simulink model "Karatsuba_Multiplier_64_Unsigned"  (R2012b)
settings: Solver=FixedStepDiscrete  SolverMode=SingleTasking  StartTime=0  StopTime=stopClock  RelTol=1e-3
libraries: xbsIndex_r4 x469
(part 1 of 3)
settings Model: Creator=UGG1  LastModifiedBy=UGG1

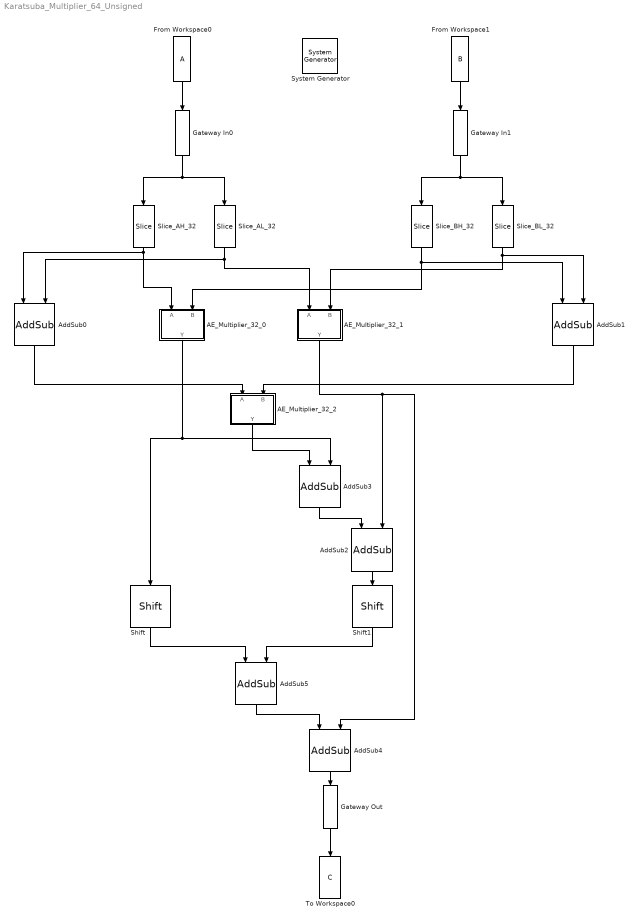
== system Karatsuba_Multiplier_64_Unsigned ==
  " System Generator" : xbsIndex_r4/ System Generator  Tag=genX  xilinxfamily=Kintex7  part=xc7k325t  speed=-3  package=fbg676  synthesis_tool=XST  clock_wrapper=Clock Enables  directory=./netlist  proj_type=Project Navigator  Synth_file=XST Defaults  Impl_file=ISE Defaults  testbench=off  simulink_period=1  sysclk_period=10  dcm_input_clock_period=10  incr_netlist=off  trim_vbits=Everywhere in SubSystem  dbl_ovrd=According to Block Masks  core_generation=According to Block Masks  run_coregen=off  deprecated_control=off  eval_field=0  block_type=sysgen
  AE_Multiplier_32_0 : Subsystem
  AE_Multiplier_32_1 : Subsystem
  AE_Multiplier_32_2 : Subsystem
  AddSub0 : xbsIndex_r4/AddSub  mode=Addition  use_carryin=off  use_carryout=off  en=off  latency=0  precision=User Defined  arith_type=Unsigned  n_bits=33  bin_pt=0  quantization=Truncate  overflow=Wrap  dbl_ovrd=off  use_behavioral_HDL=off  hw_selection=Fabric  pipelined=on  block_type=addsub
  AddSub1 : xbsIndex_r4/AddSub  mode=Addition  use_carryin=off  use_carryout=off  en=off  latency=0  precision=User Defined  arith_type=Unsigned  n_bits=33  bin_pt=0  quantization=Truncate  overflow=Wrap  dbl_ovrd=off  use_behavioral_HDL=off  hw_selection=Fabric  pipelined=on  block_type=addsub
  AddSub2 : xbsIndex_r4/AddSub  mode=Subtraction  use_carryin=off  use_carryout=off  en=off  latency=0  precision=User Defined  arith_type=Unsigned  n_bits=64  bin_pt=0  quantization=Truncate  overflow=Wrap  dbl_ovrd=off  use_behavioral_HDL=off  hw_selection=Fabric  pipelined=on  block_type=addsub
  AddSub3 : xbsIndex_r4/AddSub  mode=Subtraction  use_carryin=off  use_carryout=off  en=off  latency=0  precision=User Defined  arith_type=Unsigned  n_bits=64  bin_pt=0  quantization=Truncate  overflow=Wrap  dbl_ovrd=off  use_behavioral_HDL=off  hw_selection=Fabric  pipelined=on  block_type=addsub
  AddSub4 : xbsIndex_r4/AddSub  mode=Addition  use_carryin=off  use_carryout=off  en=off  latency=0  precision=User Defined  arith_type=Unsigned  n_bits=128  bin_pt=0  quantization=Truncate  overflow=Wrap  dbl_ovrd=off  use_behavioral_HDL=off  hw_selection=Fabric  pipelined=on  block_type=addsub
  AddSub5 : xbsIndex_r4/AddSub  mode=Addition  use_carryin=off  use_carryout=off  en=off  latency=0  precision=User Defined  arith_type=Unsigned  n_bits=128  bin_pt=0  quantization=Truncate  overflow=Wrap  dbl_ovrd=off  use_behavioral_HDL=off  hw_selection=Fabric  pipelined=on  block_type=addsub
  From Workspace0 : FromWorkspace  VariableName=A  SampleTime=0
  From Workspace1 : FromWorkspace  VariableName=B  SampleTime=0
  Gateway In0 : xbsIndex_r4/Gateway In  gui_display_data_type=Fixed-point  arith_type=Unsigned  n_bits=64  bin_pt=0  preci_type=Single  exp_width=8  frac_width=24  quantization="Round  (unbiased: +/- Inf)"  overflow=Saturate  period=1  dbl_ovrd=off  timing_constraint=None  locs_specified=off  LOCs={}  UseAsADC=off  ADCChannel='1'  inherit_from_input=off  hdl_port=on  block_type=gatewayin
  Gateway In1 : xbsIndex_r4/Gateway In  gui_display_data_type=Fixed-point  arith_type=Unsigned  n_bits=64  bin_pt=0  preci_type=Single  exp_width=8  frac_width=24  quantization="Round  (unbiased: +/- Inf)"  overflow=Saturate  period=1  dbl_ovrd=off  timing_constraint=None  locs_specified=off  LOCs={}  UseAsADC=off  ADCChannel='1'  inherit_from_input=off  hdl_port=on  block_type=gatewayin
  Gateway Out : xbsIndex_r4/Gateway Out  inherit_from_input=off  hdl_port=on  timing_constraint=None  locs_specified=off  LOCs={}  UseAsDAC=off  DACChannel='1'  block_type=gatewayout
  Shift : xbsIndex_r4/Shift  shift_dir=Left  shift_bits=64  en=off  latency=0  precision=User Defined  arith_type=Unsigned  n_bits=128  bin_pt=0  quantization=Truncate  overflow=Wrap  dbl_ovrd=off  block_type=shift
  Shift1 : xbsIndex_r4/Shift  shift_dir=Left  shift_bits=32  en=off  latency=0  precision=User Defined  arith_type=Unsigned  n_bits=128  bin_pt=0  quantization=Truncate  overflow=Wrap  dbl_ovrd=off  block_type=shift
  Slice_AH_32 : xbsIndex_r4/Slice  nbits=32  boolean_output=off  mode=Lower Bit Location + Width  bit1=0  base1=MSB of Input  bit0=32  base0=LSB of Input  dbl_ovrd=off  block_type=slice
  Slice_AL_32 : xbsIndex_r4/Slice  nbits=32  boolean_output=off  mode=Lower Bit Location + Width  bit1=0  base1=MSB of Input  bit0=0  base0=LSB of Input  dbl_ovrd=off  block_type=slice
  Slice_BH_32 : xbsIndex_r4/Slice  nbits=32  boolean_output=off  mode=Lower Bit Location + Width  bit1=0  base1=MSB of Input  bit0=32  base0=LSB of Input  dbl_ovrd=off  block_type=slice
  Slice_BL_32 : xbsIndex_r4/Slice  nbits=32  boolean_output=off  mode=Lower Bit Location + Width  bit1=0  base1=MSB of Input  bit0=0  base0=LSB of Input  dbl_ovrd=off  block_type=slice
  To Workspace0 : ToWorkspace  VariableName=C  SampleTime=-1  SaveFormat=Timeseries
  wires:
  From Workspace1/1 -> Gateway In1/1
  Gateway Out/1 -> To Workspace0/1
  From Workspace0/1 -> Gateway In0/1
  Gateway In0/1 -> Slice_AL_32/1, Slice_AH_32/1
  Gateway In1/1 -> Slice_BL_32/1, Slice_BH_32/1
  Slice_AH_32/1 -> AE_Multiplier_32_0/1(A), AddSub0/1
  Slice_BH_32/1 -> AE_Multiplier_32_0/2(B), AddSub1/1
  Slice_BL_32/1 -> AddSub1/2, AE_Multiplier_32_1/2(B)
  Slice_AL_32/1 -> AddSub0/2, AE_Multiplier_32_1/1(A)
  AddSub0/1 -> AE_Multiplier_32_2/1(A)
  AddSub1/1 -> AE_Multiplier_32_2/2(B)
  AE_Multiplier_32_2/1(Y) -> AddSub3/1
  AE_Multiplier_32_0/1(Y) -> Shift/1, AddSub3/2
  AddSub3/1 -> AddSub2/1
  AE_Multiplier_32_1/1(Y) -> AddSub4/2, AddSub2/2
  AddSub2/1 -> Shift1/1
  Shift/1 -> AddSub5/1
  Shift1/1 -> AddSub5/2
  AddSub5/1 -> AddSub4/1
  AddSub4/1 -> Gateway Out/1

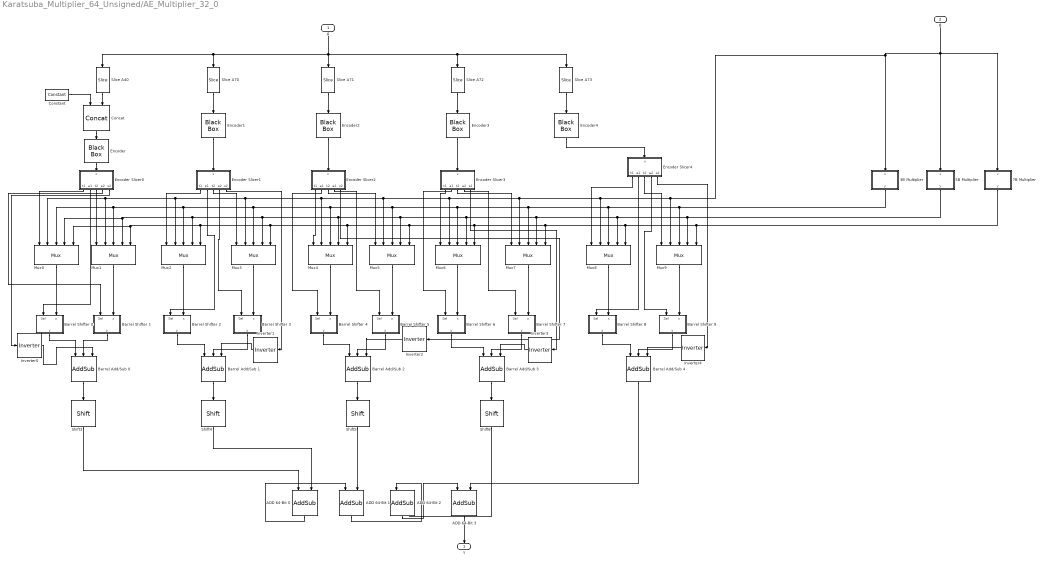
== system Karatsuba_Multiplier_64_Unsigned/AE_Multiplier_32_0 ==
  A : Inport
  B : Inport  Port=2
  3B Multiplier : Subsystem
  5B Multiplier : Subsystem
  7B Multiplier : Subsystem
  ADD 64-Bit {0..3} (4 alike) : xbsIndex_r4/AddSub  mode=Addition  use_carryin=off  use_carryout=off  en=off  latency=0  precision=User Defined  arith_type=Unsigned  n_bits=128  bin_pt=0  quantization=Truncate  overflow=Wrap  dbl_ovrd=off  use_behavioral_HDL=off  hw_selection=Fabric  pipelined=on  block_type=addsub
  Barrel Add/Sub {0..4} (5 alike) : xbsIndex_r4/AddSub  mode=Addition or Subtraction  use_carryin=off  use_carryout=off  en=off  latency=0  precision=User Defined  arith_type=Unsigned  n_bits=64  bin_pt=0  quantization=Truncate  overflow=Wrap  dbl_ovrd=off  use_behavioral_HDL=off  hw_selection=Fabric  pipelined=on  block_type=addsub
  Barrel Shifter 0 : Subsystem
  Barrel Shifter 1 : Subsystem
  Barrel Shifter 2 : Subsystem
  Barrel Shifter 3 : Subsystem
  Barrel Shifter 4 : Subsystem
  Barrel Shifter 5 : Subsystem
  Barrel Shifter 6 : Subsystem
  Barrel Shifter 7 : Subsystem
  Barrel Shifter 8 : Subsystem
  Barrel Shifter 9 : Subsystem
  Concat : xbsIndex_r4/Concat  num_inputs=2  dbl_ovrd=off  block_type=concat
  Constant : xbsIndex_r4/Constant  const=0  gui_display_data_type=Fixed-point  arith_type=Unsigned  n_bits=3  bin_pt=0  preci_type=Single  exp_width=8  frac_width=24  explicit_period=off  period=1  equ=P=C  opselect=C  inp2=PCIN>>17  opr=+  inp1=P  carry=CIN  dbl_ovrd=off  block_type=constant
  Encoder{,1..4} (5 alike) : xbsIndex_r4/Black Box  init_code=MUltiplier_Encoder_7_Bit_config  sim_method=ISE Simulator  verbose=off  block_type=blackbox2
  Encoder Slicer0 : Subsystem
  Encoder Slicer1 : Subsystem
  Encoder Slicer2 : Subsystem
  Encoder Slicer3 : Subsystem
  Encoder Slicer4 : Subsystem
  Inverter{0..4} (5 alike) : xbsIndex_r4/Inverter  en=off  latency=0  dbl_ovrd=off  block_type=inv
  Mux{0..9} (10 alike) : xbsIndex_r4/Mux  inputs=4  en=off  latency=0  precision=User Defined  arith_type=Unsigned  n_bits=38  bin_pt=0  quantization=Truncate  overflow=Wrap  dbl_ovrd=off  block_type=mux
  Shift3 : xbsIndex_r4/Shift  shift_dir=Left  shift_bits=28  en=off  latency=0  precision=User Defined  arith_type=Unsigned  n_bits=92  bin_pt=0  quantization=Truncate  overflow=Wrap  dbl_ovrd=off  block_type=shift
  Shift4 : xbsIndex_r4/Shift  shift_dir=Left  shift_bits=21  en=off  latency=0  precision=User Defined  arith_type=Unsigned  n_bits=85  bin_pt=0  quantization=Truncate  overflow=Wrap  dbl_ovrd=off  block_type=shift
  Shift5 : xbsIndex_r4/Shift  shift_dir=Left  shift_bits=14  en=off  latency=0  precision=User Defined  arith_type=Unsigned  n_bits=78  bin_pt=0  quantization=Truncate  overflow=Wrap  dbl_ovrd=off  block_type=shift
  Shift6 : xbsIndex_r4/Shift  shift_dir=Left  shift_bits=7  en=off  latency=0  precision=User Defined  arith_type=Unsigned  n_bits=71  bin_pt=0  quantization=Truncate  overflow=Wrap  dbl_ovrd=off  block_type=shift
  Slice A40 : xbsIndex_r4/Slice  nbits=4  boolean_output=off  mode=Lower Bit Location + Width  bit1=0  base1=MSB of Input  bit0=28  base0=LSB of Input  dbl_ovrd=off  block_type=slice
  Slice A70 : xbsIndex_r4/Slice  nbits=7  boolean_output=off  mode=Lower Bit Location + Width  bit1=0  base1=MSB of Input  bit0=21  base0=LSB of Input  dbl_ovrd=off  block_type=slice
  Slice A71 : xbsIndex_r4/Slice  nbits=7  boolean_output=off  mode=Lower Bit Location + Width  bit1=0  base1=MSB of Input  bit0=14  base0=LSB of Input  dbl_ovrd=off  block_type=slice
  Slice A72 : xbsIndex_r4/Slice  nbits=7  boolean_output=off  mode=Lower Bit Location + Width  bit1=0  base1=MSB of Input  bit0=7  base0=LSB of Input  dbl_ovrd=off  block_type=slice
  Slice A73 : xbsIndex_r4/Slice  nbits=7  boolean_output=off  mode=Lower Bit Location + Width  bit1=0  base1=MSB of Input  bit0=0  base0=LSB of Input  dbl_ovrd=off  block_type=slice
  Y : Outport
  wires:
  Inverter0/1 -> Barrel Add/Sub 0/3
  Encoder Slicer1/5(s2) -> Inverter1/1
  Constant/1 -> Concat/1
  Inverter1/1 -> Barrel Add/Sub 1/3
  Encoder Slicer0/5(s2) -> Inverter0/1
  Inverter4/1 -> Barrel Add/Sub 4/3
  Encoder Slicer2/5(s2) -> Inverter2/1
  Encoder Slicer3/5(s2) -> Inverter3/1
  Encoder Slicer4/5(s2) -> Inverter4/1
  Inverter3/1 -> Barrel Add/Sub 3/3
  3B Multiplier/1(y) -> Mux9/3, Mux8/3, Mux7/3, Mux6/3, Mux5/3, Mux4/3, Mux3/3, Mux2/3, Mux1/3, Mux0/3
  5B Multiplier/1(y) -> Mux9/4, Mux8/4, Mux7/4, Mux6/4, Mux5/4, Mux4/4, Mux3/4, Mux2/4, Mux1/4, Mux0/4
  7B Multiplier/1(y) -> Mux9/5, Mux8/5, Mux7/5, Mux6/5, Mux5/5, Mux4/5, Mux3/5, Mux2/5, Mux1/5, Mux0/5
  Slice A70/1 -> Encoder1/1
  Slice A71/1 -> Encoder2/1
  Slice A72/1 -> Encoder3/1
  Slice A73/1 -> Encoder4/1
  A/1 -> Slice A73/1, Slice A72/1, Slice A40/1, Slice A70/1, Slice A71/1
  ADD 64-Bit 0/1 -> ADD 64-Bit 1/1
  ADD 64-Bit 1/1 -> ADD 64-Bit 2/1
  ADD 64-Bit 2/1 -> ADD 64-Bit 3/1
  ADD 64-Bit 3/1 -> Y/1
  Encoder/1 -> Encoder Slicer0/1(x)
  Encoder1/1 -> Encoder Slicer1/1(x)
  Encoder2/1 -> Encoder Slicer2/1(x)
  Encoder3/1 -> Encoder Slicer3/1(x)
  Encoder4/1 -> Encoder Slicer4/1(x)
  B/1 -> 7B Multiplier/1(x), 5B Multiplier/1(x), 3B Multiplier/1(x), Mux9/2, Mux8/2, Mux7/2, Mux6/2, Mux4/2, Mux3/2, Mux2/2, Mux1/2, Mux0/2, Mux5/2
  Encoder Slicer0/1(t1) -> Mux0/1
  Encoder Slicer0/3(t2) -> Mux1/1
  Encoder Slicer1/1(t1) -> Mux2/1
  Encoder Slicer1/3(t2) -> Mux3/1
  Encoder Slicer2/1(t1) -> Mux4/1
  Encoder Slicer4/3(t2) -> Mux9/1
  Encoder Slicer4/1(t1) -> Mux8/1
  Encoder Slicer3/3(t2) -> Mux7/1
  Encoder Slicer3/1(t1) -> Mux6/1
  Encoder Slicer2/3(t2) -> Mux5/1
  Encoder Slicer0/2(a1) -> Barrel Shifter 0/1(Sel)
  Encoder Slicer0/4(a2) -> Barrel Shifter 1/1(Sel)
  Encoder Slicer1/2(a1) -> Barrel Shifter 2/1(Sel)
  Encoder Slicer1/4(a2) -> Barrel Shifter 3/1(Sel)
  Encoder Slicer2/2(a1) -> Barrel Shifter 4/1(Sel)
  Encoder Slicer2/4(a2) -> Barrel Shifter 5/1(Sel)
  Encoder Slicer3/2(a1) -> Barrel Shifter 6/1(Sel)
  Encoder Slicer3/4(a2) -> Barrel Shifter 7/1(Sel)
  Encoder Slicer4/2(a1) -> Barrel Shifter 8/1(Sel)
  Encoder Slicer4/4(a2) -> Barrel Shifter 9/1(Sel)
  Mux8/1 -> Barrel Shifter 8/2(x)
  Mux9/1 -> Barrel Shifter 9/2(x)
  Mux6/1 -> Barrel Shifter 6/2(x)
  Mux7/1 -> Barrel Shifter 7/2(x)
  Mux4/1 -> Barrel Shifter 4/2(x)
  Mux5/1 -> Barrel Shifter 5/2(x)
  Mux2/1 -> Barrel Shifter 2/2(x)
  Mux3/1 -> Barrel Shifter 3/2(x)
  Mux0/1 -> Barrel Shifter 0/2(x)
  Mux1/1 -> Barrel Shifter 1/2(x)
  Barrel Shifter 8/1(y) -> Barrel Add/Sub 4/1
  Barrel Shifter 9/1(y) -> Barrel Add/Sub 4/2
  Barrel Shifter 6/1(y) -> Barrel Add/Sub 3/1
  Barrel Shifter 7/1(y) -> Barrel Add/Sub 3/2
  Barrel Shifter 4/1(y) -> Barrel Add/Sub 2/1
  Barrel Shifter 5/1(y) -> Barrel Add/Sub 2/2
  Barrel Shifter 2/1(y) -> Barrel Add/Sub 1/1
  Barrel Shifter 3/1(y) -> Barrel Add/Sub 1/2
  Barrel Shifter 0/1(y) -> Barrel Add/Sub 0/1
  Barrel Shifter 1/1(y) -> Barrel Add/Sub 0/2
  Barrel Add/Sub 0/1 -> Shift3/1
  Barrel Add/Sub 1/1 -> Shift4/1
  Barrel Add/Sub 2/1 -> Shift5/1
  Barrel Add/Sub 3/1 -> Shift6/1
  Shift3/1 -> ADD 64-Bit 0/1
  Shift4/1 -> ADD 64-Bit 0/2
  Shift5/1 -> ADD 64-Bit 1/2
  Shift6/1 -> ADD 64-Bit 2/2
  Barrel Add/Sub 4/1 -> ADD 64-Bit 3/2
  Concat/1 -> Encoder/1
  Slice A40/1 -> Concat/2
  Inverter2/1 -> Barrel Add/Sub 2/3

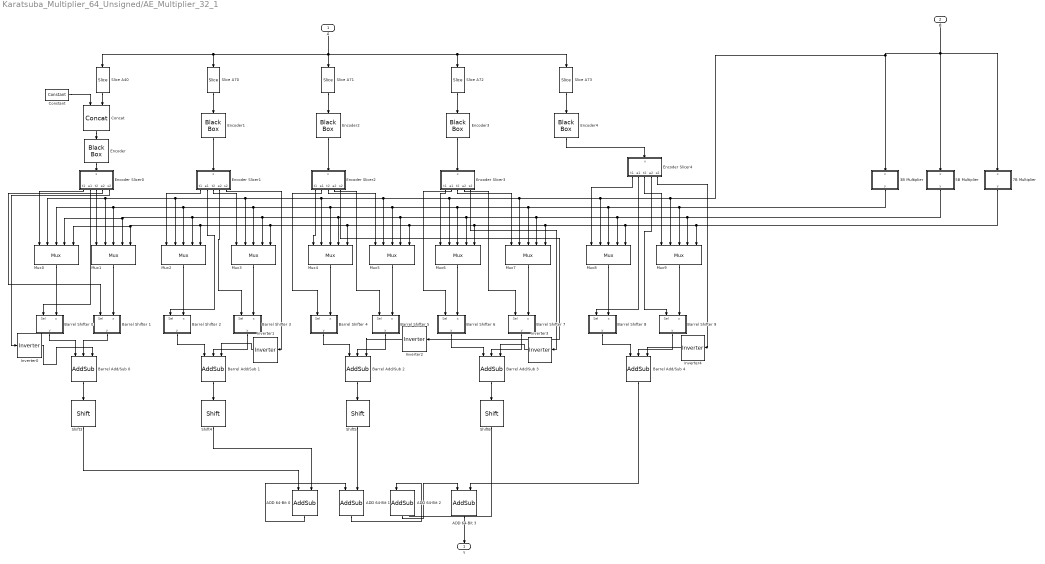
== system Karatsuba_Multiplier_64_Unsigned/AE_Multiplier_32_1 ==
  A : Inport
  B : Inport  Port=2
  3B Multiplier : Subsystem
  5B Multiplier : Subsystem
  7B Multiplier : Subsystem
  ADD 64-Bit {0..3} (4 alike) : xbsIndex_r4/AddSub  mode=Addition  use_carryin=off  use_carryout=off  en=off  latency=0  precision=User Defined  arith_type=Unsigned  n_bits=128  bin_pt=0  quantization=Truncate  overflow=Wrap  dbl_ovrd=off  use_behavioral_HDL=off  hw_selection=Fabric  pipelined=on  block_type=addsub
  Barrel Add/Sub {0..4} (5 alike) : xbsIndex_r4/AddSub  mode=Addition or Subtraction  use_carryin=off  use_carryout=off  en=off  latency=0  precision=User Defined  arith_type=Unsigned  n_bits=64  bin_pt=0  quantization=Truncate  overflow=Wrap  dbl_ovrd=off  use_behavioral_HDL=off  hw_selection=Fabric  pipelined=on  block_type=addsub
  Barrel Shifter 0 : Subsystem
  Barrel Shifter 1 : Subsystem
  Barrel Shifter 2 : Subsystem
  Barrel Shifter 3 : Subsystem
  Barrel Shifter 4 : Subsystem
  Barrel Shifter 5 : Subsystem
  Barrel Shifter 6 : Subsystem
  Barrel Shifter 7 : Subsystem
  Barrel Shifter 8 : Subsystem
  Barrel Shifter 9 : Subsystem
  Concat : xbsIndex_r4/Concat  num_inputs=2  dbl_ovrd=off  block_type=concat
  Constant : xbsIndex_r4/Constant  const=0  gui_display_data_type=Fixed-point  arith_type=Unsigned  n_bits=3  bin_pt=0  preci_type=Single  exp_width=8  frac_width=24  explicit_period=off  period=1  equ=P=C  opselect=C  inp2=PCIN>>17  opr=+  inp1=P  carry=CIN  dbl_ovrd=off  block_type=constant
  Encoder{,1..4} (5 alike) : xbsIndex_r4/Black Box  init_code=MUltiplier_Encoder_7_Bit_config  sim_method=ISE Simulator  verbose=off  block_type=blackbox2
  Encoder Slicer0 : Subsystem
  Encoder Slicer1 : Subsystem
  Encoder Slicer2 : Subsystem
  Encoder Slicer3 : Subsystem
  Encoder Slicer4 : Subsystem
  Inverter{0..4} (5 alike) : xbsIndex_r4/Inverter  en=off  latency=0  dbl_ovrd=off  block_type=inv
  Mux{0..9} (10 alike) : xbsIndex_r4/Mux  inputs=4  en=off  latency=0  precision=User Defined  arith_type=Unsigned  n_bits=38  bin_pt=0  quantization=Truncate  overflow=Wrap  dbl_ovrd=off  block_type=mux
  Shift3 : xbsIndex_r4/Shift  shift_dir=Left  shift_bits=28  en=off  latency=0  precision=User Defined  arith_type=Unsigned  n_bits=92  bin_pt=0  quantization=Truncate  overflow=Wrap  dbl_ovrd=off  block_type=shift
  Shift4 : xbsIndex_r4/Shift  shift_dir=Left  shift_bits=21  en=off  latency=0  precision=User Defined  arith_type=Unsigned  n_bits=85  bin_pt=0  quantization=Truncate  overflow=Wrap  dbl_ovrd=off  block_type=shift
  Shift5 : xbsIndex_r4/Shift  shift_dir=Left  shift_bits=14  en=off  latency=0  precision=User Defined  arith_type=Unsigned  n_bits=78  bin_pt=0  quantization=Truncate  overflow=Wrap  dbl_ovrd=off  block_type=shift
  Shift6 : xbsIndex_r4/Shift  shift_dir=Left  shift_bits=7  en=off  latency=0  precision=User Defined  arith_type=Unsigned  n_bits=71  bin_pt=0  quantization=Truncate  overflow=Wrap  dbl_ovrd=off  block_type=shift
  Slice A40 : xbsIndex_r4/Slice  nbits=4  boolean_output=off  mode=Lower Bit Location + Width  bit1=0  base1=MSB of Input  bit0=28  base0=LSB of Input  dbl_ovrd=off  block_type=slice
  Slice A70 : xbsIndex_r4/Slice  nbits=7  boolean_output=off  mode=Lower Bit Location + Width  bit1=0  base1=MSB of Input  bit0=21  base0=LSB of Input  dbl_ovrd=off  block_type=slice
  Slice A71 : xbsIndex_r4/Slice  nbits=7  boolean_output=off  mode=Lower Bit Location + Width  bit1=0  base1=MSB of Input  bit0=14  base0=LSB of Input  dbl_ovrd=off  block_type=slice
  Slice A72 : xbsIndex_r4/Slice  nbits=7  boolean_output=off  mode=Lower Bit Location + Width  bit1=0  base1=MSB of Input  bit0=7  base0=LSB of Input  dbl_ovrd=off  block_type=slice
  Slice A73 : xbsIndex_r4/Slice  nbits=7  boolean_output=off  mode=Lower Bit Location + Width  bit1=0  base1=MSB of Input  bit0=0  base0=LSB of Input  dbl_ovrd=off  block_type=slice
  Y : Outport
  wires:
  Inverter0/1 -> Barrel Add/Sub 0/3
  Encoder Slicer1/5(s2) -> Inverter1/1
  Constant/1 -> Concat/1
  Inverter1/1 -> Barrel Add/Sub 1/3
  Encoder Slicer0/5(s2) -> Inverter0/1
  Inverter4/1 -> Barrel Add/Sub 4/3
  Encoder Slicer2/5(s2) -> Inverter2/1
  Encoder Slicer3/5(s2) -> Inverter3/1
  Encoder Slicer4/5(s2) -> Inverter4/1
  Inverter3/1 -> Barrel Add/Sub 3/3
  3B Multiplier/1(y) -> Mux9/3, Mux8/3, Mux7/3, Mux6/3, Mux5/3, Mux4/3, Mux3/3, Mux2/3, Mux1/3, Mux0/3
  5B Multiplier/1(y) -> Mux9/4, Mux8/4, Mux7/4, Mux6/4, Mux5/4, Mux4/4, Mux3/4, Mux2/4, Mux1/4, Mux0/4
  7B Multiplier/1(y) -> Mux9/5, Mux8/5, Mux7/5, Mux6/5, Mux5/5, Mux4/5, Mux3/5, Mux2/5, Mux1/5, Mux0/5
  Slice A70/1 -> Encoder1/1
  Slice A71/1 -> Encoder2/1
  Slice A72/1 -> Encoder3/1
  Slice A73/1 -> Encoder4/1
  A/1 -> Slice A73/1, Slice A72/1, Slice A40/1, Slice A70/1, Slice A71/1
  ADD 64-Bit 0/1 -> ADD 64-Bit 1/1
  ADD 64-Bit 1/1 -> ADD 64-Bit 2/1
  ADD 64-Bit 2/1 -> ADD 64-Bit 3/1
  ADD 64-Bit 3/1 -> Y/1
  Encoder/1 -> Encoder Slicer0/1(x)
  Encoder1/1 -> Encoder Slicer1/1(x)
  Encoder2/1 -> Encoder Slicer2/1(x)
  Encoder3/1 -> Encoder Slicer3/1(x)
  Encoder4/1 -> Encoder Slicer4/1(x)
  B/1 -> 7B Multiplier/1(x), 5B Multiplier/1(x), 3B Multiplier/1(x), Mux9/2, Mux8/2, Mux7/2, Mux6/2, Mux4/2, Mux3/2, Mux2/2, Mux1/2, Mux0/2, Mux5/2
  Encoder Slicer0/1(t1) -> Mux0/1
  Encoder Slicer0/3(t2) -> Mux1/1
  Encoder Slicer1/1(t1) -> Mux2/1
  Encoder Slicer1/3(t2) -> Mux3/1
  Encoder Slicer2/1(t1) -> Mux4/1
  Encoder Slicer4/3(t2) -> Mux9/1
  Encoder Slicer4/1(t1) -> Mux8/1
  Encoder Slicer3/3(t2) -> Mux7/1
  Encoder Slicer3/1(t1) -> Mux6/1
  Encoder Slicer2/3(t2) -> Mux5/1
  Encoder Slicer0/2(a1) -> Barrel Shifter 0/1(Sel)
  Encoder Slicer0/4(a2) -> Barrel Shifter 1/1(Sel)
  Encoder Slicer1/2(a1) -> Barrel Shifter 2/1(Sel)
  Encoder Slicer1/4(a2) -> Barrel Shifter 3/1(Sel)
  Encoder Slicer2/2(a1) -> Barrel Shifter 4/1(Sel)
  Encoder Slicer2/4(a2) -> Barrel Shifter 5/1(Sel)
  Encoder Slicer3/2(a1) -> Barrel Shifter 6/1(Sel)
  Encoder Slicer3/4(a2) -> Barrel Shifter 7/1(Sel)
  Encoder Slicer4/2(a1) -> Barrel Shifter 8/1(Sel)
  Encoder Slicer4/4(a2) -> Barrel Shifter 9/1(Sel)
  Mux8/1 -> Barrel Shifter 8/2(x)
  Mux9/1 -> Barrel Shifter 9/2(x)
  Mux6/1 -> Barrel Shifter 6/2(x)
  Mux7/1 -> Barrel Shifter 7/2(x)
  Mux4/1 -> Barrel Shifter 4/2(x)
  Mux5/1 -> Barrel Shifter 5/2(x)
  Mux2/1 -> Barrel Shifter 2/2(x)
  Mux3/1 -> Barrel Shifter 3/2(x)
  Mux0/1 -> Barrel Shifter 0/2(x)
  Mux1/1 -> Barrel Shifter 1/2(x)
  Barrel Shifter 8/1(y) -> Barrel Add/Sub 4/1
  Barrel Shifter 9/1(y) -> Barrel Add/Sub 4/2
  Barrel Shifter 6/1(y) -> Barrel Add/Sub 3/1
  Barrel Shifter 7/1(y) -> Barrel Add/Sub 3/2
  Barrel Shifter 4/1(y) -> Barrel Add/Sub 2/1
  Barrel Shifter 5/1(y) -> Barrel Add/Sub 2/2
  Barrel Shifter 2/1(y) -> Barrel Add/Sub 1/1
  Barrel Shifter 3/1(y) -> Barrel Add/Sub 1/2
  Barrel Shifter 0/1(y) -> Barrel Add/Sub 0/1
  Barrel Shifter 1/1(y) -> Barrel Add/Sub 0/2
  Barrel Add/Sub 0/1 -> Shift3/1
  Barrel Add/Sub 1/1 -> Shift4/1
  Barrel Add/Sub 2/1 -> Shift5/1
  Barrel Add/Sub 3/1 -> Shift6/1
  Shift3/1 -> ADD 64-Bit 0/1
  Shift4/1 -> ADD 64-Bit 0/2
  Shift5/1 -> ADD 64-Bit 1/2
  Shift6/1 -> ADD 64-Bit 2/2
  Barrel Add/Sub 4/1 -> ADD 64-Bit 3/2
  Concat/1 -> Encoder/1
  Slice A40/1 -> Concat/2
  Inverter2/1 -> Barrel Add/Sub 2/3

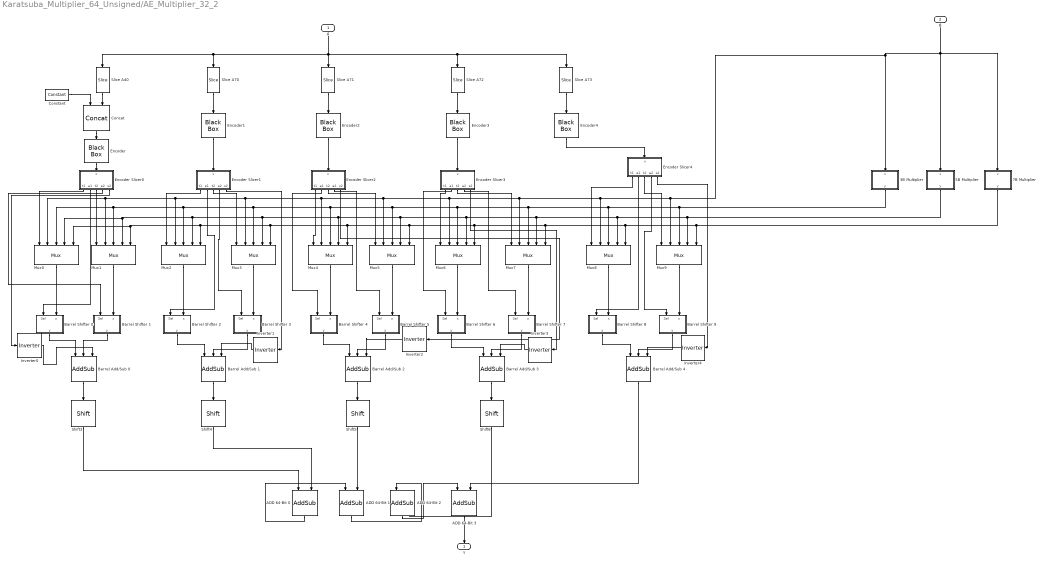
== system Karatsuba_Multiplier_64_Unsigned/AE_Multiplier_32_2 ==
  A : Inport
  B : Inport  Port=2
  3B Multiplier : Subsystem
  5B Multiplier : Subsystem
  7B Multiplier : Subsystem
  ADD 64-Bit {0..3} (4 alike) : xbsIndex_r4/AddSub  mode=Addition  use_carryin=off  use_carryout=off  en=off  latency=0  precision=User Defined  arith_type=Unsigned  n_bits=128  bin_pt=0  quantization=Truncate  overflow=Wrap  dbl_ovrd=off  use_behavioral_HDL=off  hw_selection=Fabric  pipelined=on  block_type=addsub
  Barrel Add/Sub {0..4} (5 alike) : xbsIndex_r4/AddSub  mode=Addition or Subtraction  use_carryin=off  use_carryout=off  en=off  latency=0  precision=User Defined  arith_type=Unsigned  n_bits=64  bin_pt=0  quantization=Truncate  overflow=Wrap  dbl_ovrd=off  use_behavioral_HDL=off  hw_selection=Fabric  pipelined=on  block_type=addsub
  Barrel Shifter 0 : Subsystem
  Barrel Shifter 1 : Subsystem
  Barrel Shifter 2 : Subsystem
  Barrel Shifter 3 : Subsystem
  Barrel Shifter 4 : Subsystem
  Barrel Shifter 5 : Subsystem
  Barrel Shifter 6 : Subsystem
  Barrel Shifter 7 : Subsystem
  Barrel Shifter 8 : Subsystem
  Barrel Shifter 9 : Subsystem
  Concat : xbsIndex_r4/Concat  num_inputs=2  dbl_ovrd=off  block_type=concat
  Constant : xbsIndex_r4/Constant  const=0  gui_display_data_type=Fixed-point  arith_type=Unsigned  n_bits=3  bin_pt=0  preci_type=Single  exp_width=8  frac_width=24  explicit_period=off  period=1  equ=P=C  opselect=C  inp2=PCIN>>17  opr=+  inp1=P  carry=CIN  dbl_ovrd=off  block_type=constant
  Encoder{,1..4} (5 alike) : xbsIndex_r4/Black Box  init_code=MUltiplier_Encoder_7_Bit_config  sim_method=ISE Simulator  verbose=off  block_type=blackbox2
  Encoder Slicer0 : Subsystem
  Encoder Slicer1 : Subsystem
  Encoder Slicer2 : Subsystem
  Encoder Slicer3 : Subsystem
  Encoder Slicer4 : Subsystem
  Inverter{0..4} (5 alike) : xbsIndex_r4/Inverter  en=off  latency=0  dbl_ovrd=off  block_type=inv
  Mux{0..9} (10 alike) : xbsIndex_r4/Mux  inputs=4  en=off  latency=0  precision=User Defined  arith_type=Unsigned  n_bits=38  bin_pt=0  quantization=Truncate  overflow=Wrap  dbl_ovrd=off  block_type=mux
  Shift3 : xbsIndex_r4/Shift  shift_dir=Left  shift_bits=28  en=off  latency=0  precision=User Defined  arith_type=Unsigned  n_bits=92  bin_pt=0  quantization=Truncate  overflow=Wrap  dbl_ovrd=off  block_type=shift
  Shift4 : xbsIndex_r4/Shift  shift_dir=Left  shift_bits=21  en=off  latency=0  precision=User Defined  arith_type=Unsigned  n_bits=85  bin_pt=0  quantization=Truncate  overflow=Wrap  dbl_ovrd=off  block_type=shift
  Shift5 : xbsIndex_r4/Shift  shift_dir=Left  shift_bits=14  en=off  latency=0  precision=User Defined  arith_type=Unsigned  n_bits=78  bin_pt=0  quantization=Truncate  overflow=Wrap  dbl_ovrd=off  block_type=shift
  Shift6 : xbsIndex_r4/Shift  shift_dir=Left  shift_bits=7  en=off  latency=0  precision=User Defined  arith_type=Unsigned  n_bits=71  bin_pt=0  quantization=Truncate  overflow=Wrap  dbl_ovrd=off  block_type=shift
  Slice A40 : xbsIndex_r4/Slice  nbits=4  boolean_output=off  mode=Lower Bit Location + Width  bit1=0  base1=MSB of Input  bit0=28  base0=LSB of Input  dbl_ovrd=off  block_type=slice
  Slice A70 : xbsIndex_r4/Slice  nbits=7  boolean_output=off  mode=Lower Bit Location + Width  bit1=0  base1=MSB of Input  bit0=21  base0=LSB of Input  dbl_ovrd=off  block_type=slice
  Slice A71 : xbsIndex_r4/Slice  nbits=7  boolean_output=off  mode=Lower Bit Location + Width  bit1=0  base1=MSB of Input  bit0=14  base0=LSB of Input  dbl_ovrd=off  block_type=slice
  Slice A72 : xbsIndex_r4/Slice  nbits=7  boolean_output=off  mode=Lower Bit Location + Width  bit1=0  base1=MSB of Input  bit0=7  base0=LSB of Input  dbl_ovrd=off  block_type=slice
  Slice A73 : xbsIndex_r4/Slice  nbits=7  boolean_output=off  mode=Lower Bit Location + Width  bit1=0  base1=MSB of Input  bit0=0  base0=LSB of Input  dbl_ovrd=off  block_type=slice
  Y : Outport
  wires:
  Inverter0/1 -> Barrel Add/Sub 0/3
  Encoder Slicer1/5(s2) -> Inverter1/1
  Constant/1 -> Concat/1
  Inverter1/1 -> Barrel Add/Sub 1/3
  Encoder Slicer0/5(s2) -> Inverter0/1
  Inverter4/1 -> Barrel Add/Sub 4/3
  Encoder Slicer2/5(s2) -> Inverter2/1
  Encoder Slicer3/5(s2) -> Inverter3/1
  Encoder Slicer4/5(s2) -> Inverter4/1
  Inverter3/1 -> Barrel Add/Sub 3/3
  3B Multiplier/1(y) -> Mux9/3, Mux8/3, Mux7/3, Mux6/3, Mux5/3, Mux4/3, Mux3/3, Mux2/3, Mux1/3, Mux0/3
  5B Multiplier/1(y) -> Mux9/4, Mux8/4, Mux7/4, Mux6/4, Mux5/4, Mux4/4, Mux3/4, Mux2/4, Mux1/4, Mux0/4
  7B Multiplier/1(y) -> Mux9/5, Mux8/5, Mux7/5, Mux6/5, Mux5/5, Mux4/5, Mux3/5, Mux2/5, Mux1/5, Mux0/5
  Slice A70/1 -> Encoder1/1
  Slice A71/1 -> Encoder2/1
  Slice A72/1 -> Encoder3/1
  Slice A73/1 -> Encoder4/1
  A/1 -> Slice A73/1, Slice A72/1, Slice A40/1, Slice A70/1, Slice A71/1
  ADD 64-Bit 0/1 -> ADD 64-Bit 1/1
  ADD 64-Bit 1/1 -> ADD 64-Bit 2/1
  ADD 64-Bit 2/1 -> ADD 64-Bit 3/1
  ADD 64-Bit 3/1 -> Y/1
  Encoder/1 -> Encoder Slicer0/1(x)
  Encoder1/1 -> Encoder Slicer1/1(x)
  Encoder2/1 -> Encoder Slicer2/1(x)
  Encoder3/1 -> Encoder Slicer3/1(x)
  Encoder4/1 -> Encoder Slicer4/1(x)
  B/1 -> 7B Multiplier/1(x), 5B Multiplier/1(x), 3B Multiplier/1(x), Mux9/2, Mux8/2, Mux7/2, Mux6/2, Mux4/2, Mux3/2, Mux2/2, Mux1/2, Mux0/2, Mux5/2
  Encoder Slicer0/1(t1) -> Mux0/1
  Encoder Slicer0/3(t2) -> Mux1/1
  Encoder Slicer1/1(t1) -> Mux2/1
  Encoder Slicer1/3(t2) -> Mux3/1
  Encoder Slicer2/1(t1) -> Mux4/1
  Encoder Slicer4/3(t2) -> Mux9/1
  Encoder Slicer4/1(t1) -> Mux8/1
  Encoder Slicer3/3(t2) -> Mux7/1
  Encoder Slicer3/1(t1) -> Mux6/1
  Encoder Slicer2/3(t2) -> Mux5/1
  Encoder Slicer0/2(a1) -> Barrel Shifter 0/1(Sel)
  Encoder Slicer0/4(a2) -> Barrel Shifter 1/1(Sel)
  Encoder Slicer1/2(a1) -> Barrel Shifter 2/1(Sel)
  Encoder Slicer1/4(a2) -> Barrel Shifter 3/1(Sel)
  Encoder Slicer2/2(a1) -> Barrel Shifter 4/1(Sel)
  Encoder Slicer2/4(a2) -> Barrel Shifter 5/1(Sel)
  Encoder Slicer3/2(a1) -> Barrel Shifter 6/1(Sel)
  Encoder Slicer3/4(a2) -> Barrel Shifter 7/1(Sel)
  Encoder Slicer4/2(a1) -> Barrel Shifter 8/1(Sel)
  Encoder Slicer4/4(a2) -> Barrel Shifter 9/1(Sel)
  Mux8/1 -> Barrel Shifter 8/2(x)
  Mux9/1 -> Barrel Shifter 9/2(x)
  Mux6/1 -> Barrel Shifter 6/2(x)
  Mux7/1 -> Barrel Shifter 7/2(x)
  Mux4/1 -> Barrel Shifter 4/2(x)
  Mux5/1 -> Barrel Shifter 5/2(x)
  Mux2/1 -> Barrel Shifter 2/2(x)
  Mux3/1 -> Barrel Shifter 3/2(x)
  Mux0/1 -> Barrel Shifter 0/2(x)
  Mux1/1 -> Barrel Shifter 1/2(x)
  Barrel Shifter 8/1(y) -> Barrel Add/Sub 4/1
  Barrel Shifter 9/1(y) -> Barrel Add/Sub 4/2
  Barrel Shifter 6/1(y) -> Barrel Add/Sub 3/1
  Barrel Shifter 7/1(y) -> Barrel Add/Sub 3/2
  Barrel Shifter 4/1(y) -> Barrel Add/Sub 2/1
  Barrel Shifter 5/1(y) -> Barrel Add/Sub 2/2
  Barrel Shifter 2/1(y) -> Barrel Add/Sub 1/1
  Barrel Shifter 3/1(y) -> Barrel Add/Sub 1/2
  Barrel Shifter 0/1(y) -> Barrel Add/Sub 0/1
  Barrel Shifter 1/1(y) -> Barrel Add/Sub 0/2
  Barrel Add/Sub 0/1 -> Shift3/1
  Barrel Add/Sub 1/1 -> Shift4/1
  Barrel Add/Sub 2/1 -> Shift5/1
  Barrel Add/Sub 3/1 -> Shift6/1
  Shift3/1 -> ADD 64-Bit 0/1
  Shift4/1 -> ADD 64-Bit 0/2
  Shift5/1 -> ADD 64-Bit 1/2
  Shift6/1 -> ADD 64-Bit 2/2
  Barrel Add/Sub 4/1 -> ADD 64-Bit 3/2
  Concat/1 -> Encoder/1
  Slice A40/1 -> Concat/2
  Inverter2/1 -> Barrel Add/Sub 2/3

== system Karatsuba_Multiplier_64_Unsigned/AE_Multiplier_32_0/3B Multiplier ==
  x : Inport
  AddSub : xbsIndex_r4/AddSub  mode=Addition  use_carryin=off  use_carryout=off  en=off  latency=0  precision=User Defined  arith_type=Unsigned  n_bits=64  bin_pt=0  quantization=Truncate  overflow=Wrap  dbl_ovrd=off  use_behavioral_HDL=off  hw_selection=Fabric  pipelined=on  block_type=addsub
  Shift : xbsIndex_r4/Shift  shift_dir=Left  shift_bits=1  en=off  latency=0  precision=User Defined  arith_type=Unsigned  n_bits=64  bin_pt=0  quantization=Truncate  overflow=Wrap  dbl_ovrd=off  block_type=shift
  y : Outport
  wires:
  x/1 -> Shift/1, AddSub/2
  AddSub/1 -> y/1
  Shift/1 -> AddSub/1

== system Karatsuba_Multiplier_64_Unsigned/AE_Multiplier_32_0/5B Multiplier ==
  x : Inport
  AddSub1 : xbsIndex_r4/AddSub  mode=Addition  use_carryin=off  use_carryout=off  en=off  latency=0  precision=User Defined  arith_type=Unsigned  n_bits=64  bin_pt=0  quantization=Truncate  overflow=Wrap  dbl_ovrd=off  use_behavioral_HDL=off  hw_selection=Fabric  pipelined=on  block_type=addsub
  Shift1 : xbsIndex_r4/Shift  shift_dir=Left  shift_bits=2  en=off  latency=0  precision=User Defined  arith_type=Unsigned  n_bits=64  bin_pt=0  quantization=Truncate  overflow=Wrap  dbl_ovrd=off  block_type=shift
  y : Outport
  wires:
  x/1 -> AddSub1/2, Shift1/1
  Shift1/1 -> AddSub1/1
  AddSub1/1 -> y/1

== system Karatsuba_Multiplier_64_Unsigned/AE_Multiplier_32_0/7B Multiplier ==
  x : Inport
  AddSub2 : xbsIndex_r4/AddSub  mode=Subtraction  use_carryin=off  use_carryout=off  en=off  latency=0  precision=User Defined  arith_type=Unsigned  n_bits=64  bin_pt=0  quantization=Truncate  overflow=Wrap  dbl_ovrd=off  use_behavioral_HDL=off  hw_selection=Fabric  pipelined=on  block_type=addsub
  Shift2 : xbsIndex_r4/Shift  shift_dir=Left  shift_bits=3  en=off  latency=0  precision=User Defined  arith_type=Unsigned  n_bits=64  bin_pt=0  quantization=Truncate  overflow=Wrap  dbl_ovrd=off  block_type=shift
  y : Outport
  wires:
  AddSub2/1 -> y/1
  Shift2/1 -> AddSub2/1
  x/1 -> Shift2/1, AddSub2/2

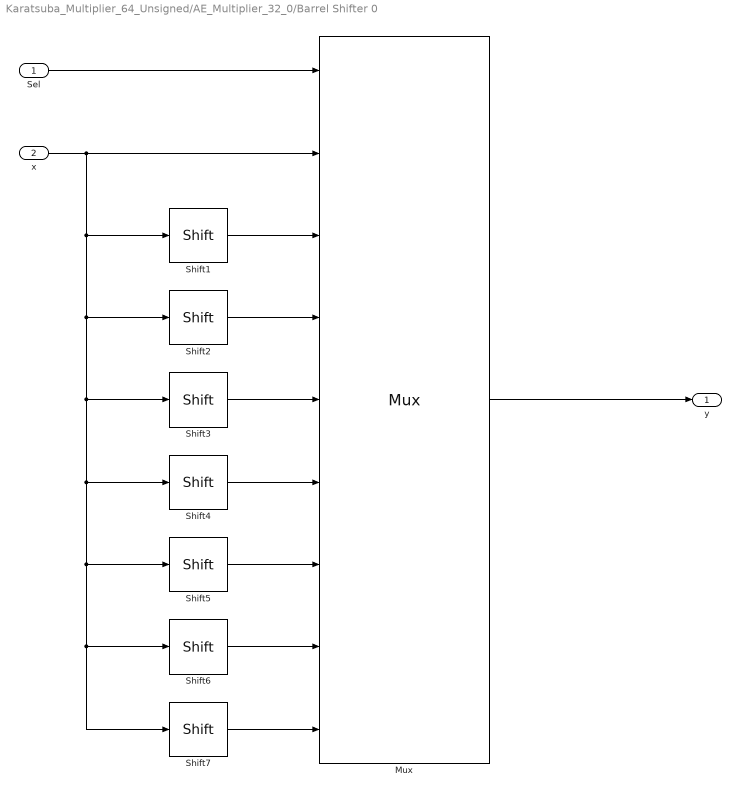
== system Karatsuba_Multiplier_64_Unsigned/AE_Multiplier_32_0/Barrel Shifter 0 ==
  Sel : Inport
  x : Inport  Port=2
  Mux : xbsIndex_r4/Mux  inputs=8  en=off  latency=0  precision=Full  arith_type=Unsigned  n_bits=17  bin_pt=0  quantization=Truncate  overflow=Wrap  dbl_ovrd=off  block_type=mux
  Shift1 : xbsIndex_r4/Shift  shift_dir=Left  shift_bits=1  en=off  latency=0  precision=User Defined  arith_type=Unsigned  n_bits=64  bin_pt=0  quantization=Truncate  overflow=Wrap  dbl_ovrd=off  block_type=shift
  Shift2 : xbsIndex_r4/Shift  shift_dir=Left  shift_bits=2  en=off  latency=0  precision=User Defined  arith_type=Unsigned  n_bits=64  bin_pt=0  quantization=Truncate  overflow=Wrap  dbl_ovrd=off  block_type=shift
  Shift3 : xbsIndex_r4/Shift  shift_dir=Left  shift_bits=3  en=off  latency=0  precision=User Defined  arith_type="Signed  (2's comp)"  n_bits=64  bin_pt=0  quantization=Truncate  overflow=Wrap  dbl_ovrd=off  block_type=shift
  Shift4 : xbsIndex_r4/Shift  shift_dir=Left  shift_bits=4  en=off  latency=0  precision=User Defined  arith_type=Unsigned  n_bits=64  bin_pt=0  quantization=Truncate  overflow=Wrap  dbl_ovrd=off  block_type=shift
  Shift5 : xbsIndex_r4/Shift  shift_dir=Left  shift_bits=5  en=off  latency=0  precision=User Defined  arith_type=Unsigned  n_bits=43  bin_pt=0  quantization=Truncate  overflow=Wrap  dbl_ovrd=off  block_type=shift
  Shift6 : xbsIndex_r4/Shift  shift_dir=Left  shift_bits=6  en=off  latency=0  precision=User Defined  arith_type=Unsigned  n_bits=64  bin_pt=0  quantization=Truncate  overflow=Wrap  dbl_ovrd=off  block_type=shift
  Shift7 : xbsIndex_r4/Shift  shift_dir=Left  shift_bits=7  en=off  latency=0  precision=User Defined  arith_type=Unsigned  n_bits=64  bin_pt=0  quantization=Truncate  overflow=Wrap  dbl_ovrd=off  block_type=shift
  y : Outport
  wires:
  Mux/1 -> y/1
  Sel/1 -> Mux/1
  x/1 -> Shift1/1, Shift2/1, Shift3/1, Shift4/1, Shift5/1, Shift6/1, Shift7/1, Mux/2
  Shift1/1 -> Mux/3
  Shift2/1 -> Mux/4
  Shift3/1 -> Mux/5
  Shift4/1 -> Mux/6
  Shift5/1 -> Mux/7
  Shift6/1 -> Mux/8
  Shift7/1 -> Mux/9

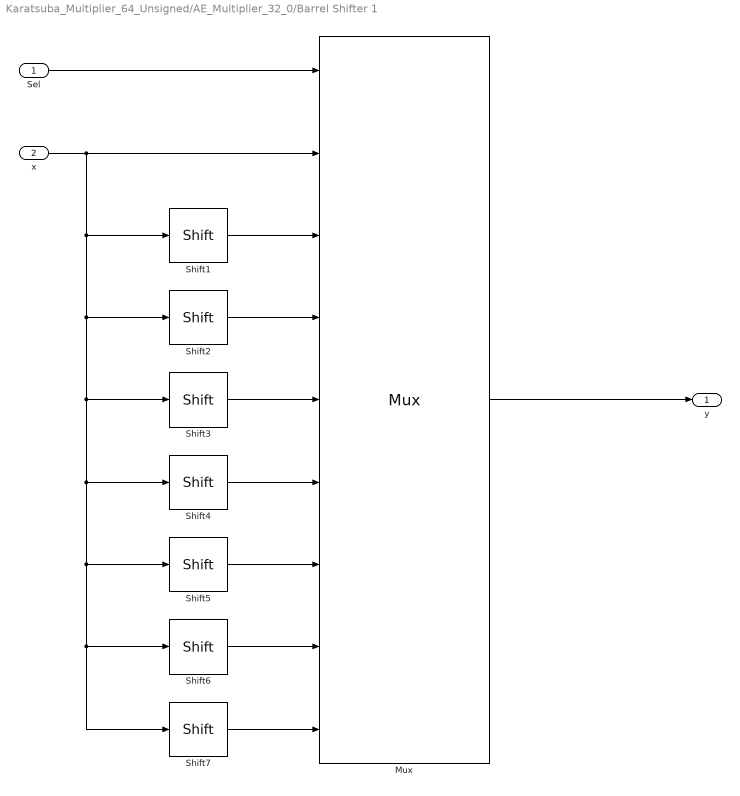
== system Karatsuba_Multiplier_64_Unsigned/AE_Multiplier_32_0/Barrel Shifter 1 ==
  Sel : Inport
  x : Inport  Port=2
  Mux : xbsIndex_r4/Mux  inputs=8  en=off  latency=0  precision=Full  arith_type=Unsigned  n_bits=17  bin_pt=0  quantization=Truncate  overflow=Wrap  dbl_ovrd=off  block_type=mux
  Shift1 : xbsIndex_r4/Shift  shift_dir=Left  shift_bits=1  en=off  latency=0  precision=User Defined  arith_type=Unsigned  n_bits=64  bin_pt=0  quantization=Truncate  overflow=Wrap  dbl_ovrd=off  block_type=shift
  Shift2 : xbsIndex_r4/Shift  shift_dir=Left  shift_bits=2  en=off  latency=0  precision=User Defined  arith_type=Unsigned  n_bits=64  bin_pt=0  quantization=Truncate  overflow=Wrap  dbl_ovrd=off  block_type=shift
  Shift3 : xbsIndex_r4/Shift  shift_dir=Left  shift_bits=3  en=off  latency=0  precision=User Defined  arith_type="Signed  (2's comp)"  n_bits=64  bin_pt=0  quantization=Truncate  overflow=Wrap  dbl_ovrd=off  block_type=shift
  Shift4 : xbsIndex_r4/Shift  shift_dir=Left  shift_bits=4  en=off  latency=0  precision=User Defined  arith_type=Unsigned  n_bits=64  bin_pt=0  quantization=Truncate  overflow=Wrap  dbl_ovrd=off  block_type=shift
  Shift5 : xbsIndex_r4/Shift  shift_dir=Left  shift_bits=5  en=off  latency=0  precision=User Defined  arith_type=Unsigned  n_bits=43  bin_pt=0  quantization=Truncate  overflow=Wrap  dbl_ovrd=off  block_type=shift
  Shift6 : xbsIndex_r4/Shift  shift_dir=Left  shift_bits=6  en=off  latency=0  precision=User Defined  arith_type=Unsigned  n_bits=64  bin_pt=0  quantization=Truncate  overflow=Wrap  dbl_ovrd=off  block_type=shift
  Shift7 : xbsIndex_r4/Shift  shift_dir=Left  shift_bits=7  en=off  latency=0  precision=User Defined  arith_type=Unsigned  n_bits=64  bin_pt=0  quantization=Truncate  overflow=Wrap  dbl_ovrd=off  block_type=shift
  y : Outport
  wires:
  Mux/1 -> y/1
  Sel/1 -> Mux/1
  x/1 -> Shift1/1, Shift2/1, Shift3/1, Shift4/1, Shift5/1, Shift6/1, Shift7/1, Mux/2
  Shift1/1 -> Mux/3
  Shift2/1 -> Mux/4
  Shift3/1 -> Mux/5
  Shift4/1 -> Mux/6
  Shift5/1 -> Mux/7
  Shift6/1 -> Mux/8
  Shift7/1 -> Mux/9

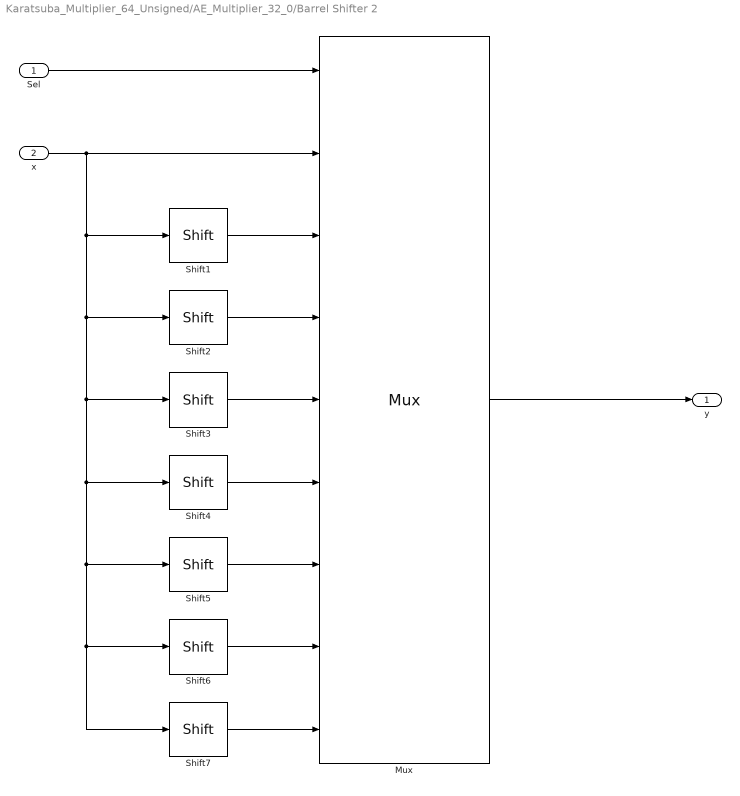
== system Karatsuba_Multiplier_64_Unsigned/AE_Multiplier_32_0/Barrel Shifter 2 ==
  Sel : Inport
  x : Inport  Port=2
  Mux : xbsIndex_r4/Mux  inputs=8  en=off  latency=0  precision=Full  arith_type=Unsigned  n_bits=17  bin_pt=0  quantization=Truncate  overflow=Wrap  dbl_ovrd=off  block_type=mux
  Shift1 : xbsIndex_r4/Shift  shift_dir=Left  shift_bits=1  en=off  latency=0  precision=User Defined  arith_type=Unsigned  n_bits=64  bin_pt=0  quantization=Truncate  overflow=Wrap  dbl_ovrd=off  block_type=shift
  Shift2 : xbsIndex_r4/Shift  shift_dir=Left  shift_bits=2  en=off  latency=0  precision=User Defined  arith_type=Unsigned  n_bits=64  bin_pt=0  quantization=Truncate  overflow=Wrap  dbl_ovrd=off  block_type=shift
  Shift3 : xbsIndex_r4/Shift  shift_dir=Left  shift_bits=3  en=off  latency=0  precision=User Defined  arith_type="Signed  (2's comp)"  n_bits=64  bin_pt=0  quantization=Truncate  overflow=Wrap  dbl_ovrd=off  block_type=shift
  Shift4 : xbsIndex_r4/Shift  shift_dir=Left  shift_bits=4  en=off  latency=0  precision=User Defined  arith_type=Unsigned  n_bits=64  bin_pt=0  quantization=Truncate  overflow=Wrap  dbl_ovrd=off  block_type=shift
  Shift5 : xbsIndex_r4/Shift  shift_dir=Left  shift_bits=5  en=off  latency=0  precision=User Defined  arith_type=Unsigned  n_bits=43  bin_pt=0  quantization=Truncate  overflow=Wrap  dbl_ovrd=off  block_type=shift
  Shift6 : xbsIndex_r4/Shift  shift_dir=Left  shift_bits=6  en=off  latency=0  precision=User Defined  arith_type=Unsigned  n_bits=64  bin_pt=0  quantization=Truncate  overflow=Wrap  dbl_ovrd=off  block_type=shift
  Shift7 : xbsIndex_r4/Shift  shift_dir=Left  shift_bits=7  en=off  latency=0  precision=User Defined  arith_type=Unsigned  n_bits=64  bin_pt=0  quantization=Truncate  overflow=Wrap  dbl_ovrd=off  block_type=shift
  y : Outport
  wires:
  Mux/1 -> y/1
  Sel/1 -> Mux/1
  x/1 -> Shift1/1, Shift2/1, Shift3/1, Shift4/1, Shift5/1, Shift6/1, Shift7/1, Mux/2
  Shift1/1 -> Mux/3
  Shift2/1 -> Mux/4
  Shift3/1 -> Mux/5
  Shift4/1 -> Mux/6
  Shift5/1 -> Mux/7
  Shift6/1 -> Mux/8
  Shift7/1 -> Mux/9

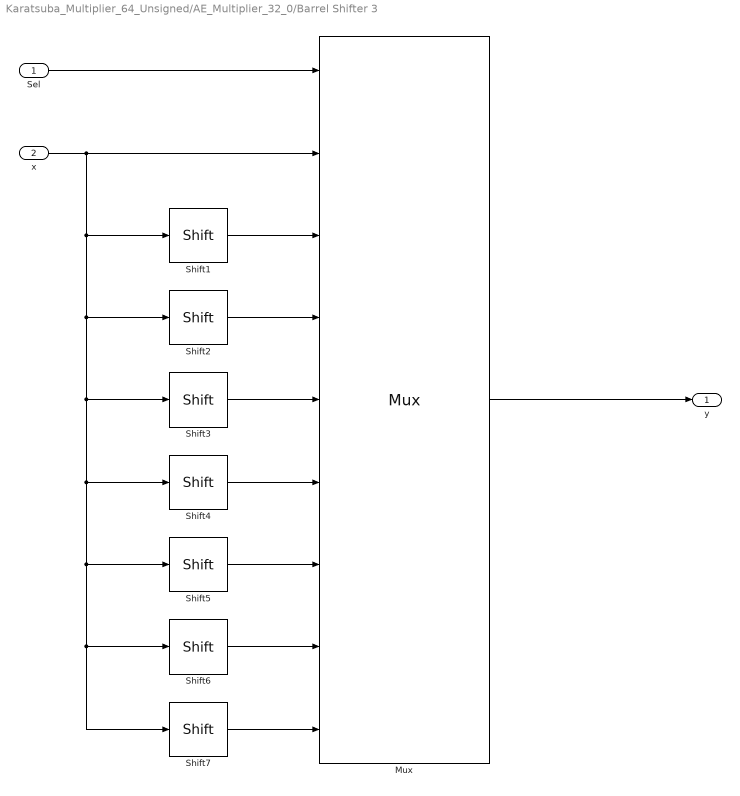
== system Karatsuba_Multiplier_64_Unsigned/AE_Multiplier_32_0/Barrel Shifter 3 ==
  Sel : Inport
  x : Inport  Port=2
  Mux : xbsIndex_r4/Mux  inputs=8  en=off  latency=0  precision=Full  arith_type=Unsigned  n_bits=17  bin_pt=0  quantization=Truncate  overflow=Wrap  dbl_ovrd=off  block_type=mux
  Shift1 : xbsIndex_r4/Shift  shift_dir=Left  shift_bits=1  en=off  latency=0  precision=User Defined  arith_type=Unsigned  n_bits=64  bin_pt=0  quantization=Truncate  overflow=Wrap  dbl_ovrd=off  block_type=shift
  Shift2 : xbsIndex_r4/Shift  shift_dir=Left  shift_bits=2  en=off  latency=0  precision=User Defined  arith_type=Unsigned  n_bits=64  bin_pt=0  quantization=Truncate  overflow=Wrap  dbl_ovrd=off  block_type=shift
  Shift3 : xbsIndex_r4/Shift  shift_dir=Left  shift_bits=3  en=off  latency=0  precision=User Defined  arith_type="Signed  (2's comp)"  n_bits=64  bin_pt=0  quantization=Truncate  overflow=Wrap  dbl_ovrd=off  block_type=shift
  Shift4 : xbsIndex_r4/Shift  shift_dir=Left  shift_bits=4  en=off  latency=0  precision=User Defined  arith_type=Unsigned  n_bits=64  bin_pt=0  quantization=Truncate  overflow=Wrap  dbl_ovrd=off  block_type=shift
  Shift5 : xbsIndex_r4/Shift  shift_dir=Left  shift_bits=5  en=off  latency=0  precision=User Defined  arith_type=Unsigned  n_bits=43  bin_pt=0  quantization=Truncate  overflow=Wrap  dbl_ovrd=off  block_type=shift
  Shift6 : xbsIndex_r4/Shift  shift_dir=Left  shift_bits=6  en=off  latency=0  precision=User Defined  arith_type=Unsigned  n_bits=64  bin_pt=0  quantization=Truncate  overflow=Wrap  dbl_ovrd=off  block_type=shift
  Shift7 : xbsIndex_r4/Shift  shift_dir=Left  shift_bits=7  en=off  latency=0  precision=User Defined  arith_type=Unsigned  n_bits=64  bin_pt=0  quantization=Truncate  overflow=Wrap  dbl_ovrd=off  block_type=shift
  y : Outport
  wires:
  Mux/1 -> y/1
  Sel/1 -> Mux/1
  x/1 -> Shift1/1, Shift2/1, Shift3/1, Shift4/1, Shift5/1, Shift6/1, Shift7/1, Mux/2
  Shift1/1 -> Mux/3
  Shift2/1 -> Mux/4
  Shift3/1 -> Mux/5
  Shift4/1 -> Mux/6
  Shift5/1 -> Mux/7
  Shift6/1 -> Mux/8
  Shift7/1 -> Mux/9

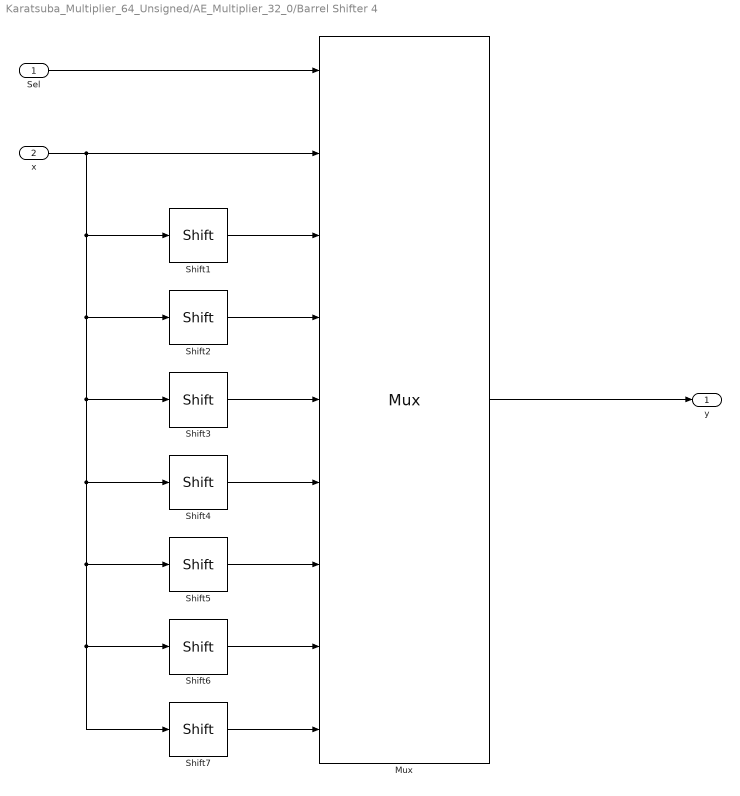
== system Karatsuba_Multiplier_64_Unsigned/AE_Multiplier_32_0/Barrel Shifter 4 ==
  Sel : Inport
  x : Inport  Port=2
  Mux : xbsIndex_r4/Mux  inputs=8  en=off  latency=0  precision=Full  arith_type=Unsigned  n_bits=17  bin_pt=0  quantization=Truncate  overflow=Wrap  dbl_ovrd=off  block_type=mux
  Shift1 : xbsIndex_r4/Shift  shift_dir=Left  shift_bits=1  en=off  latency=0  precision=User Defined  arith_type=Unsigned  n_bits=64  bin_pt=0  quantization=Truncate  overflow=Wrap  dbl_ovrd=off  block_type=shift
  Shift2 : xbsIndex_r4/Shift  shift_dir=Left  shift_bits=2  en=off  latency=0  precision=User Defined  arith_type=Unsigned  n_bits=64  bin_pt=0  quantization=Truncate  overflow=Wrap  dbl_ovrd=off  block_type=shift
  Shift3 : xbsIndex_r4/Shift  shift_dir=Left  shift_bits=3  en=off  latency=0  precision=User Defined  arith_type="Signed  (2's comp)"  n_bits=64  bin_pt=0  quantization=Truncate  overflow=Wrap  dbl_ovrd=off  block_type=shift
  Shift4 : xbsIndex_r4/Shift  shift_dir=Left  shift_bits=4  en=off  latency=0  precision=User Defined  arith_type=Unsigned  n_bits=64  bin_pt=0  quantization=Truncate  overflow=Wrap  dbl_ovrd=off  block_type=shift
  Shift5 : xbsIndex_r4/Shift  shift_dir=Left  shift_bits=5  en=off  latency=0  precision=User Defined  arith_type=Unsigned  n_bits=43  bin_pt=0  quantization=Truncate  overflow=Wrap  dbl_ovrd=off  block_type=shift
  Shift6 : xbsIndex_r4/Shift  shift_dir=Left  shift_bits=6  en=off  latency=0  precision=User Defined  arith_type=Unsigned  n_bits=64  bin_pt=0  quantization=Truncate  overflow=Wrap  dbl_ovrd=off  block_type=shift
  Shift7 : xbsIndex_r4/Shift  shift_dir=Left  shift_bits=7  en=off  latency=0  precision=User Defined  arith_type=Unsigned  n_bits=64  bin_pt=0  quantization=Truncate  overflow=Wrap  dbl_ovrd=off  block_type=shift
  y : Outport
  wires:
  Mux/1 -> y/1
  Sel/1 -> Mux/1
  x/1 -> Shift1/1, Shift2/1, Shift3/1, Shift4/1, Shift5/1, Shift6/1, Shift7/1, Mux/2
  Shift1/1 -> Mux/3
  Shift2/1 -> Mux/4
  Shift3/1 -> Mux/5
  Shift4/1 -> Mux/6
  Shift5/1 -> Mux/7
  Shift6/1 -> Mux/8
  Shift7/1 -> Mux/9

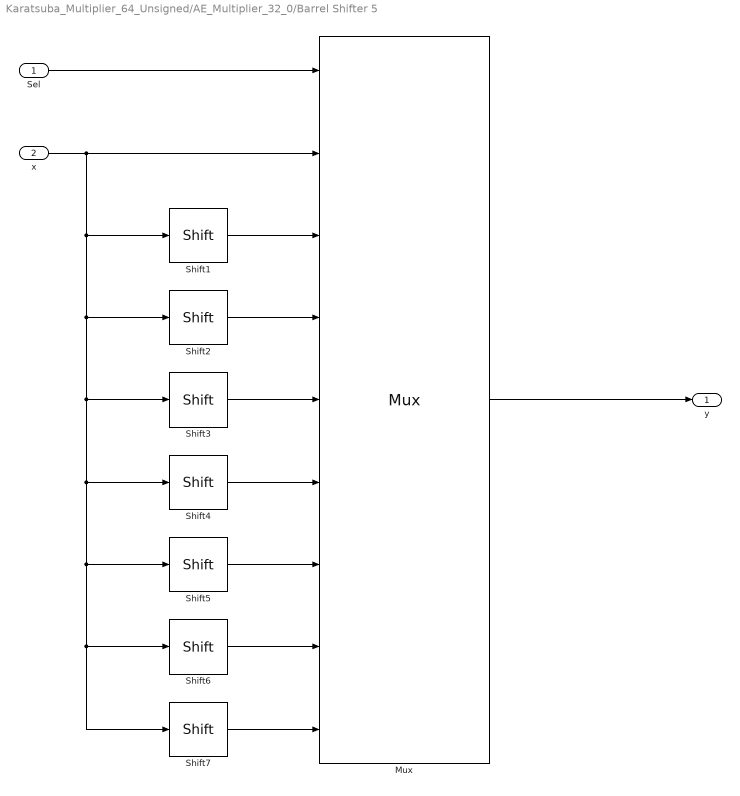
== system Karatsuba_Multiplier_64_Unsigned/AE_Multiplier_32_0/Barrel Shifter 5 ==
  Sel : Inport
  x : Inport  Port=2
  Mux : xbsIndex_r4/Mux  inputs=8  en=off  latency=0  precision=Full  arith_type=Unsigned  n_bits=17  bin_pt=0  quantization=Truncate  overflow=Wrap  dbl_ovrd=off  block_type=mux
  Shift1 : xbsIndex_r4/Shift  shift_dir=Left  shift_bits=1  en=off  latency=0  precision=User Defined  arith_type=Unsigned  n_bits=64  bin_pt=0  quantization=Truncate  overflow=Wrap  dbl_ovrd=off  block_type=shift
  Shift2 : xbsIndex_r4/Shift  shift_dir=Left  shift_bits=2  en=off  latency=0  precision=User Defined  arith_type=Unsigned  n_bits=64  bin_pt=0  quantization=Truncate  overflow=Wrap  dbl_ovrd=off  block_type=shift
  Shift3 : xbsIndex_r4/Shift  shift_dir=Left  shift_bits=3  en=off  latency=0  precision=User Defined  arith_type="Signed  (2's comp)"  n_bits=64  bin_pt=0  quantization=Truncate  overflow=Wrap  dbl_ovrd=off  block_type=shift
  Shift4 : xbsIndex_r4/Shift  shift_dir=Left  shift_bits=4  en=off  latency=0  precision=User Defined  arith_type=Unsigned  n_bits=64  bin_pt=0  quantization=Truncate  overflow=Wrap  dbl_ovrd=off  block_type=shift
  Shift5 : xbsIndex_r4/Shift  shift_dir=Left  shift_bits=5  en=off  latency=0  precision=User Defined  arith_type=Unsigned  n_bits=43  bin_pt=0  quantization=Truncate  overflow=Wrap  dbl_ovrd=off  block_type=shift
  Shift6 : xbsIndex_r4/Shift  shift_dir=Left  shift_bits=6  en=off  latency=0  precision=User Defined  arith_type=Unsigned  n_bits=64  bin_pt=0  quantization=Truncate  overflow=Wrap  dbl_ovrd=off  block_type=shift
  Shift7 : xbsIndex_r4/Shift  shift_dir=Left  shift_bits=7  en=off  latency=0  precision=User Defined  arith_type=Unsigned  n_bits=64  bin_pt=0  quantization=Truncate  overflow=Wrap  dbl_ovrd=off  block_type=shift
  y : Outport
  wires:
  Mux/1 -> y/1
  Sel/1 -> Mux/1
  x/1 -> Shift1/1, Shift2/1, Shift3/1, Shift4/1, Shift5/1, Shift6/1, Shift7/1, Mux/2
  Shift1/1 -> Mux/3
  Shift2/1 -> Mux/4
  Shift3/1 -> Mux/5
  Shift4/1 -> Mux/6
  Shift5/1 -> Mux/7
  Shift6/1 -> Mux/8
  Shift7/1 -> Mux/9

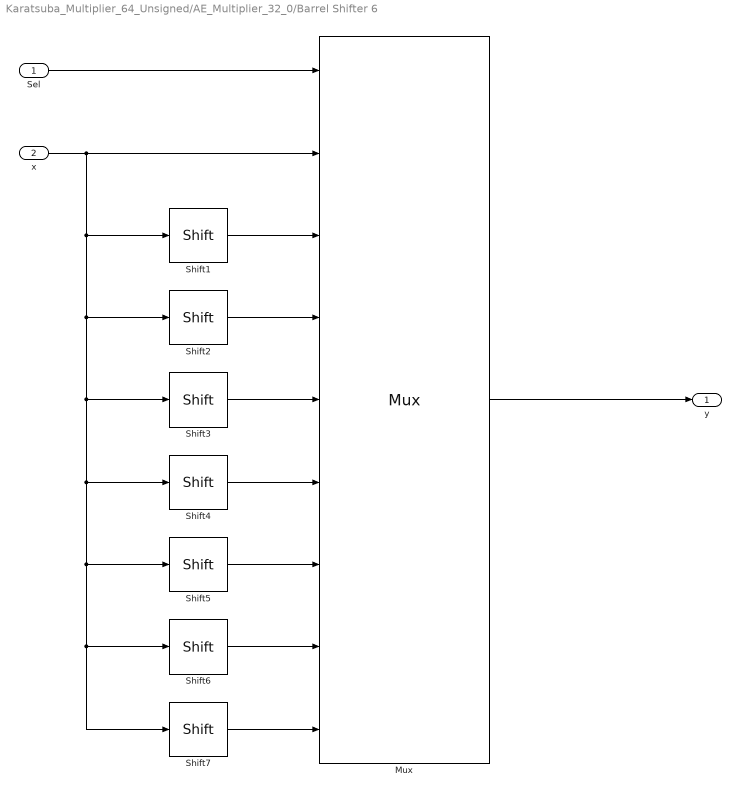
== system Karatsuba_Multiplier_64_Unsigned/AE_Multiplier_32_0/Barrel Shifter 6 ==
  Sel : Inport
  x : Inport  Port=2
  Mux : xbsIndex_r4/Mux  inputs=8  en=off  latency=0  precision=Full  arith_type=Unsigned  n_bits=17  bin_pt=0  quantization=Truncate  overflow=Wrap  dbl_ovrd=off  block_type=mux
  Shift1 : xbsIndex_r4/Shift  shift_dir=Left  shift_bits=1  en=off  latency=0  precision=User Defined  arith_type=Unsigned  n_bits=64  bin_pt=0  quantization=Truncate  overflow=Wrap  dbl_ovrd=off  block_type=shift
  Shift2 : xbsIndex_r4/Shift  shift_dir=Left  shift_bits=2  en=off  latency=0  precision=User Defined  arith_type=Unsigned  n_bits=64  bin_pt=0  quantization=Truncate  overflow=Wrap  dbl_ovrd=off  block_type=shift
  Shift3 : xbsIndex_r4/Shift  shift_dir=Left  shift_bits=3  en=off  latency=0  precision=User Defined  arith_type="Signed  (2's comp)"  n_bits=64  bin_pt=0  quantization=Truncate  overflow=Wrap  dbl_ovrd=off  block_type=shift
  Shift4 : xbsIndex_r4/Shift  shift_dir=Left  shift_bits=4  en=off  latency=0  precision=User Defined  arith_type=Unsigned  n_bits=64  bin_pt=0  quantization=Truncate  overflow=Wrap  dbl_ovrd=off  block_type=shift
  Shift5 : xbsIndex_r4/Shift  shift_dir=Left  shift_bits=5  en=off  latency=0  precision=User Defined  arith_type=Unsigned  n_bits=43  bin_pt=0  quantization=Truncate  overflow=Wrap  dbl_ovrd=off  block_type=shift
  Shift6 : xbsIndex_r4/Shift  shift_dir=Left  shift_bits=6  en=off  latency=0  precision=User Defined  arith_type=Unsigned  n_bits=64  bin_pt=0  quantization=Truncate  overflow=Wrap  dbl_ovrd=off  block_type=shift
  Shift7 : xbsIndex_r4/Shift  shift_dir=Left  shift_bits=7  en=off  latency=0  precision=User Defined  arith_type=Unsigned  n_bits=64  bin_pt=0  quantization=Truncate  overflow=Wrap  dbl_ovrd=off  block_type=shift
  y : Outport
  wires:
  Mux/1 -> y/1
  Sel/1 -> Mux/1
  x/1 -> Shift1/1, Shift2/1, Shift3/1, Shift4/1, Shift5/1, Shift6/1, Shift7/1, Mux/2
  Shift1/1 -> Mux/3
  Shift2/1 -> Mux/4
  Shift3/1 -> Mux/5
  Shift4/1 -> Mux/6
  Shift5/1 -> Mux/7
  Shift6/1 -> Mux/8
  Shift7/1 -> Mux/9

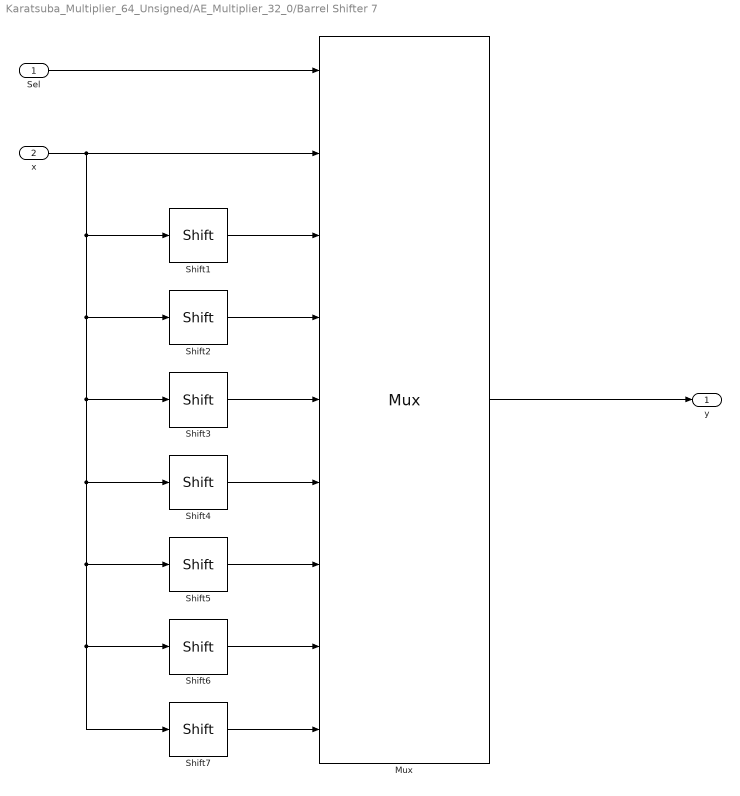
== system Karatsuba_Multiplier_64_Unsigned/AE_Multiplier_32_0/Barrel Shifter 7 ==
  Sel : Inport
  x : Inport  Port=2
  Mux : xbsIndex_r4/Mux  inputs=8  en=off  latency=0  precision=Full  arith_type=Unsigned  n_bits=17  bin_pt=0  quantization=Truncate  overflow=Wrap  dbl_ovrd=off  block_type=mux
  Shift1 : xbsIndex_r4/Shift  shift_dir=Left  shift_bits=1  en=off  latency=0  precision=User Defined  arith_type=Unsigned  n_bits=64  bin_pt=0  quantization=Truncate  overflow=Wrap  dbl_ovrd=off  block_type=shift
  Shift2 : xbsIndex_r4/Shift  shift_dir=Left  shift_bits=2  en=off  latency=0  precision=User Defined  arith_type=Unsigned  n_bits=64  bin_pt=0  quantization=Truncate  overflow=Wrap  dbl_ovrd=off  block_type=shift
  Shift3 : xbsIndex_r4/Shift  shift_dir=Left  shift_bits=3  en=off  latency=0  precision=User Defined  arith_type="Signed  (2's comp)"  n_bits=64  bin_pt=0  quantization=Truncate  overflow=Wrap  dbl_ovrd=off  block_type=shift
  Shift4 : xbsIndex_r4/Shift  shift_dir=Left  shift_bits=4  en=off  latency=0  precision=User Defined  arith_type=Unsigned  n_bits=64  bin_pt=0  quantization=Truncate  overflow=Wrap  dbl_ovrd=off  block_type=shift
  Shift5 : xbsIndex_r4/Shift  shift_dir=Left  shift_bits=5  en=off  latency=0  precision=User Defined  arith_type=Unsigned  n_bits=43  bin_pt=0  quantization=Truncate  overflow=Wrap  dbl_ovrd=off  block_type=shift
  Shift6 : xbsIndex_r4/Shift  shift_dir=Left  shift_bits=6  en=off  latency=0  precision=User Defined  arith_type=Unsigned  n_bits=64  bin_pt=0  quantization=Truncate  overflow=Wrap  dbl_ovrd=off  block_type=shift
  Shift7 : xbsIndex_r4/Shift  shift_dir=Left  shift_bits=7  en=off  latency=0  precision=User Defined  arith_type=Unsigned  n_bits=64  bin_pt=0  quantization=Truncate  overflow=Wrap  dbl_ovrd=off  block_type=shift
  y : Outport
  wires:
  Mux/1 -> y/1
  Sel/1 -> Mux/1
  x/1 -> Shift1/1, Shift2/1, Shift3/1, Shift4/1, Shift5/1, Shift6/1, Shift7/1, Mux/2
  Shift1/1 -> Mux/3
  Shift2/1 -> Mux/4
  Shift3/1 -> Mux/5
  Shift4/1 -> Mux/6
  Shift5/1 -> Mux/7
  Shift6/1 -> Mux/8
  Shift7/1 -> Mux/9

== system Karatsuba_Multiplier_64_Unsigned/AE_Multiplier_32_0/Barrel Shifter 8 ==
  Sel : Inport
  x : Inport  Port=2
  Mux : xbsIndex_r4/Mux  inputs=8  en=off  latency=0  precision=Full  arith_type=Unsigned  n_bits=17  bin_pt=0  quantization=Truncate  overflow=Wrap  dbl_ovrd=off  block_type=mux
  Shift1 : xbsIndex_r4/Shift  shift_dir=Left  shift_bits=1  en=off  latency=0  precision=User Defined  arith_type=Unsigned  n_bits=64  bin_pt=0  quantization=Truncate  overflow=Wrap  dbl_ovrd=off  block_type=shift
  Shift2 : xbsIndex_r4/Shift  shift_dir=Left  shift_bits=2  en=off  latency=0  precision=User Defined  arith_type=Unsigned  n_bits=64  bin_pt=0  quantization=Truncate  overflow=Wrap  dbl_ovrd=off  block_type=shift
  Shift3 : xbsIndex_r4/Shift  shift_dir=Left  shift_bits=3  en=off  latency=0  precision=User Defined  arith_type="Signed  (2's comp)"  n_bits=64  bin_pt=0  quantization=Truncate  overflow=Wrap  dbl_ovrd=off  block_type=shift
  Shift4 : xbsIndex_r4/Shift  shift_dir=Left  shift_bits=4  en=off  latency=0  precision=User Defined  arith_type=Unsigned  n_bits=64  bin_pt=0  quantization=Truncate  overflow=Wrap  dbl_ovrd=off  block_type=shift
  Shift5 : xbsIndex_r4/Shift  shift_dir=Left  shift_bits=5  en=off  latency=0  precision=User Defined  arith_type=Unsigned  n_bits=43  bin_pt=0  quantization=Truncate  overflow=Wrap  dbl_ovrd=off  block_type=shift
  Shift6 : xbsIndex_r4/Shift  shift_dir=Left  shift_bits=6  en=off  latency=0  precision=User Defined  arith_type=Unsigned  n_bits=64  bin_pt=0  quantization=Truncate  overflow=Wrap  dbl_ovrd=off  block_type=shift
  Shift7 : xbsIndex_r4/Shift  shift_dir=Left  shift_bits=7  en=off  latency=0  precision=User Defined  arith_type=Unsigned  n_bits=64  bin_pt=0  quantization=Truncate  overflow=Wrap  dbl_ovrd=off  block_type=shift
  y : Outport
  wires:
  Mux/1 -> y/1
  Sel/1 -> Mux/1
  x/1 -> Shift1/1, Shift2/1, Shift3/1, Shift4/1, Shift5/1, Shift6/1, Shift7/1, Mux/2
  Shift1/1 -> Mux/3
  Shift2/1 -> Mux/4
  Shift3/1 -> Mux/5
  Shift4/1 -> Mux/6
  Shift5/1 -> Mux/7
  Shift6/1 -> Mux/8
  Shift7/1 -> Mux/9
